simulink model "c00013M_harness"  (R2018a)
settings: Solver=FixedStepAuto  StartTime=0.0  StopTime=300  FixedStep=0.1  RelTol=1e-3
undefined symbols (not defined in the file): A1, hmax, PriorityTank, R1, R2, sigbuilder_block, TempThreshold
(part 8 of 93)

== system c00013M_harness/M022 ==
  note: VALUES
      | ---------------------------------
      | ControlType = 1 | 2 | 3
      | FillTank = 0 | 1
      | EmptyTank = 0 | 1
      | ManualReference between 0 and 1
      | Tempreature between 0 and 100
      | EmergencyButton = 0 | 1
      | LiquidLevel between 0 and 1 (hmax)
  note: Inputs For Tank2
  note: NAMES
      | --------------------------------------------
      | CT1 = ControlType Tank 1
      | F1 = Fill Tank 1
      | E1 = Empty Tank 1
      | MR1 = Manual Reference Tank1
      | T1 = Temperature Tank 1
      | EB1 = Emergency Button Tank 1
      | LL1 = Liquid Level 1
  note: Inputs For Tank3
  note: Inputs For Tank1
  CT1 : Inport
  T1 : Inport  Port=2
  EB1 : Inport  Port=3
  CT2 : Inport  Port=4
  F2 : Inport  Port=5
  E2 : Inport  Port=6
  MR2 : Inport  Port=7
  T2 : Inport  Port=8
  EB2 : Inport  Port=9
  CT3 : Inport  Port=10
  T3 : Inport  Port=11
  EB3 : Inport  Port=12
  Tank1 : Subsystem
  Tank2 : Subsystem
  Tank3 : Subsystem
  LL1 : Outport
  LL2 : Outport  Port=2
  LL3 : Outport  Port=3
  wires:
  EB1/1 -> Tank1/3(EB1)
  Tank2/1(LL2) -> LL2/1, Tank3/5(LL2), Tank1/4(LL2)
  Tank3/1(LL3) -> LL3/1, Tank2/8(LL3), Tank1/5(LL3)
  EB2/1 -> Tank2/6(EB2)
  CT2/1 -> Tank2/1(CT2)
  T1/1 -> Tank1/2(T1)
  Tank1/1(LL1) -> LL1/1, Tank3/4(LL1), Tank2/7(LL1)
  F2/1 -> Tank2/2(F2)
  E2/1 -> Tank2/3(E2)
  T2/1 -> Tank2/5(T2)
  CT3/1 -> Tank3/1(CT3)
  EB3/1 -> Tank3/3(EB3)
  T3/1 -> Tank3/2(T3)
  CT1/1 -> Tank1/1(CT1)
  MR2/1 -> Tank2/4(MR2)

== system c00013M_harness/M023 ==
  note: VALUES
      | ---------------------------------
      | ControlType = 1 | 2 | 3
      | FillTank = 0 | 1
      | EmptyTank = 0 | 1
      | ManualReference between 0 and 1
      | Tempreature between 0 and 100
      | EmergencyButton = 0 | 1
      | LiquidLevel between 0 and 1 (hmax)
  note: Inputs For Tank2
  note: NAMES
      | --------------------------------------------
      | CT1 = ControlType Tank 1
      | F1 = Fill Tank 1
      | E1 = Empty Tank 1
      | MR1 = Manual Reference Tank1
      | T1 = Temperature Tank 1
      | EB1 = Emergency Button Tank 1
      | LL1 = Liquid Level 1
  note: Inputs For Tank3
  note: Inputs For Tank1
  CT1 : Inport
  T1 : Inport  Port=2
  EB1 : Inport  Port=3
  CT2 : Inport  Port=4
  F2 : Inport  Port=5
  E2 : Inport  Port=6
  MR2 : Inport  Port=7
  T2 : Inport  Port=8
  EB2 : Inport  Port=9
  CT3 : Inport  Port=10
  T3 : Inport  Port=11
  EB3 : Inport  Port=12
  Tank1 : Subsystem
  Tank2 : Subsystem
  Tank3 : Subsystem
  LL1 : Outport
  LL2 : Outport  Port=2
  LL3 : Outport  Port=3
  wires:
  EB1/1 -> Tank1/3(EB1)
  Tank2/1(LL2) -> LL2/1, Tank3/5(LL2), Tank1/4(LL2)
  Tank3/1(LL3) -> LL3/1, Tank2/8(LL3), Tank1/5(LL3)
  EB2/1 -> Tank2/6(EB2)
  CT2/1 -> Tank2/1(CT2)
  T1/1 -> Tank1/2(T1)
  Tank1/1(LL1) -> LL1/1, Tank3/4(LL1), Tank2/7(LL1)
  F2/1 -> Tank2/2(F2)
  E2/1 -> Tank2/3(E2)
  T2/1 -> Tank2/5(T2)
  CT3/1 -> Tank3/1(CT3)
  EB3/1 -> Tank3/3(EB3)
  T3/1 -> Tank3/2(T3)
  CT1/1 -> Tank1/1(CT1)
  MR2/1 -> Tank2/4(MR2)

== system c00013M_harness/M024 ==
  note: VALUES
      | ---------------------------------
      | ControlType = 1 | 2 | 3
      | FillTank = 0 | 1
      | EmptyTank = 0 | 1
      | ManualReference between 0 and 1
      | Tempreature between 0 and 100
      | EmergencyButton = 0 | 1
      | LiquidLevel between 0 and 1 (hmax)
  note: Inputs For Tank2
  note: NAMES
      | --------------------------------------------
      | CT1 = ControlType Tank 1
      | F1 = Fill Tank 1
      | E1 = Empty Tank 1
      | MR1 = Manual Reference Tank1
      | T1 = Temperature Tank 1
      | EB1 = Emergency Button Tank 1
      | LL1 = Liquid Level 1
  note: Inputs For Tank3
  note: Inputs For Tank1
  CT1 : Inport
  T1 : Inport  Port=2
  EB1 : Inport  Port=3
  CT2 : Inport  Port=4
  F2 : Inport  Port=5
  E2 : Inport  Port=6
  MR2 : Inport  Port=7
  T2 : Inport  Port=8
  EB2 : Inport  Port=9
  CT3 : Inport  Port=10
  T3 : Inport  Port=11
  EB3 : Inport  Port=12
  Tank1 : Subsystem
  Tank2 : Subsystem
  Tank3 : Subsystem
  LL1 : Outport
  LL2 : Outport  Port=2
  LL3 : Outport  Port=3
  wires:
  EB1/1 -> Tank1/3(EB1)
  Tank2/1(LL2) -> LL2/1, Tank3/5(LL2), Tank1/4(LL2)
  Tank3/1(LL3) -> LL3/1, Tank2/8(LL3), Tank1/5(LL3)
  EB2/1 -> Tank2/6(EB2)
  CT2/1 -> Tank2/1(CT2)
  T1/1 -> Tank1/2(T1)
  Tank1/1(LL1) -> LL1/1, Tank3/4(LL1), Tank2/7(LL1)
  F2/1 -> Tank2/2(F2)
  E2/1 -> Tank2/3(E2)
  T2/1 -> Tank2/5(T2)
  CT3/1 -> Tank3/1(CT3)
  EB3/1 -> Tank3/3(EB3)
  T3/1 -> Tank3/2(T3)
  CT1/1 -> Tank1/1(CT1)
  MR2/1 -> Tank2/4(MR2)

== system c00013M_harness/M025 ==
  note: VALUES
      | ---------------------------------
      | ControlType = 1 | 2 | 3
      | FillTank = 0 | 1
      | EmptyTank = 0 | 1
      | ManualReference between 0 and 1
      | Tempreature between 0 and 100
      | EmergencyButton = 0 | 1
      | LiquidLevel between 0 and 1 (hmax)
  note: Inputs For Tank2
  note: NAMES
      | --------------------------------------------
      | CT1 = ControlType Tank 1
      | F1 = Fill Tank 1
      | E1 = Empty Tank 1
      | MR1 = Manual Reference Tank1
      | T1 = Temperature Tank 1
      | EB1 = Emergency Button Tank 1
      | LL1 = Liquid Level 1
  note: Inputs For Tank3
  note: Inputs For Tank1
  CT1 : Inport
  T1 : Inport  Port=2
  EB1 : Inport  Port=3
  CT2 : Inport  Port=4
  F2 : Inport  Port=5
  E2 : Inport  Port=6
  MR2 : Inport  Port=7
  T2 : Inport  Port=8
  EB2 : Inport  Port=9
  CT3 : Inport  Port=10
  T3 : Inport  Port=11
  EB3 : Inport  Port=12
  Tank1 : Subsystem
  Tank2 : Subsystem
  Tank3 : Subsystem
  LL1 : Outport
  LL2 : Outport  Port=2
  LL3 : Outport  Port=3
  wires:
  EB1/1 -> Tank1/3(EB1)
  Tank2/1(LL2) -> LL2/1, Tank3/5(LL2), Tank1/4(LL2)
  Tank3/1(LL3) -> LL3/1, Tank2/8(LL3), Tank1/5(LL3)
  EB2/1 -> Tank2/6(EB2)
  CT2/1 -> Tank2/1(CT2)
  T1/1 -> Tank1/2(T1)
  Tank1/1(LL1) -> LL1/1, Tank3/4(LL1), Tank2/7(LL1)
  F2/1 -> Tank2/2(F2)
  E2/1 -> Tank2/3(E2)
  T2/1 -> Tank2/5(T2)
  CT3/1 -> Tank3/1(CT3)
  EB3/1 -> Tank3/3(EB3)
  T3/1 -> Tank3/2(T3)
  CT1/1 -> Tank1/1(CT1)
  MR2/1 -> Tank2/4(MR2)

== system c00013M_harness/M026 ==
  note: VALUES
      | ---------------------------------
      | ControlType = 1 | 2 | 3
      | FillTank = 0 | 1
      | EmptyTank = 0 | 1
      | ManualReference between 0 and 1
      | Tempreature between 0 and 100
      | EmergencyButton = 0 | 1
      | LiquidLevel between 0 and 1 (hmax)
  note: Inputs For Tank2
  note: NAMES
      | --------------------------------------------
      | CT1 = ControlType Tank 1
      | F1 = Fill Tank 1
      | E1 = Empty Tank 1
      | MR1 = Manual Reference Tank1
      | T1 = Temperature Tank 1
      | EB1 = Emergency Button Tank 1
      | LL1 = Liquid Level 1
  note: Inputs For Tank3
  note: Inputs For Tank1
  CT1 : Inport
  T1 : Inport  Port=2
  EB1 : Inport  Port=3
  CT2 : Inport  Port=4
  F2 : Inport  Port=5
  E2 : Inport  Port=6
  MR2 : Inport  Port=7
  T2 : Inport  Port=8
  EB2 : Inport  Port=9
  CT3 : Inport  Port=10
  T3 : Inport  Port=11
  EB3 : Inport  Port=12
  Tank1 : Subsystem
  Tank2 : Subsystem
  Tank3 : Subsystem
  LL1 : Outport
  LL2 : Outport  Port=2
  LL3 : Outport  Port=3
  wires:
  EB1/1 -> Tank1/3(EB1)
  Tank2/1(LL2) -> LL2/1, Tank3/5(LL2), Tank1/4(LL2)
  Tank3/1(LL3) -> LL3/1, Tank2/8(LL3), Tank1/5(LL3)
  EB2/1 -> Tank2/6(EB2)
  CT2/1 -> Tank2/1(CT2)
  T1/1 -> Tank1/2(T1)
  Tank1/1(LL1) -> LL1/1, Tank3/4(LL1), Tank2/7(LL1)
  F2/1 -> Tank2/2(F2)
  E2/1 -> Tank2/3(E2)
  T2/1 -> Tank2/5(T2)
  CT3/1 -> Tank3/1(CT3)
  EB3/1 -> Tank3/3(EB3)
  T3/1 -> Tank3/2(T3)
  CT1/1 -> Tank1/1(CT1)
  MR2/1 -> Tank2/4(MR2)

== system c00013M_harness/M027 ==
  note: VALUES
      | ---------------------------------
      | ControlType = 1 | 2 | 3
      | FillTank = 0 | 1
      | EmptyTank = 0 | 1
      | ManualReference between 0 and 1
      | Tempreature between 0 and 100
      | EmergencyButton = 0 | 1
      | LiquidLevel between 0 and 1 (hmax)
  note: Inputs For Tank2
  note: NAMES
      | --------------------------------------------
      | CT1 = ControlType Tank 1
      | F1 = Fill Tank 1
      | E1 = Empty Tank 1
      | MR1 = Manual Reference Tank1
      | T1 = Temperature Tank 1
      | EB1 = Emergency Button Tank 1
      | LL1 = Liquid Level 1
  note: Inputs For Tank3
  note: Inputs For Tank1
  CT1 : Inport
  T1 : Inport  Port=2
  EB1 : Inport  Port=3
  CT2 : Inport  Port=4
  F2 : Inport  Port=5
  E2 : Inport  Port=6
  MR2 : Inport  Port=7
  T2 : Inport  Port=8
  EB2 : Inport  Port=9
  CT3 : Inport  Port=10
  T3 : Inport  Port=11
  EB3 : Inport  Port=12
  Tank1 : Subsystem
  Tank2 : Subsystem
  Tank3 : Subsystem
  LL1 : Outport
  LL2 : Outport  Port=2
  LL3 : Outport  Port=3
  wires:
  EB1/1 -> Tank1/3(EB1)
  Tank2/1(LL2) -> LL2/1, Tank3/5(LL2), Tank1/4(LL2)
  Tank3/1(LL3) -> LL3/1, Tank2/8(LL3), Tank1/5(LL3)
  EB2/1 -> Tank2/6(EB2)
  CT2/1 -> Tank2/1(CT2)
  T1/1 -> Tank1/2(T1)
  Tank1/1(LL1) -> LL1/1, Tank3/4(LL1), Tank2/7(LL1)
  F2/1 -> Tank2/2(F2)
  E2/1 -> Tank2/3(E2)
  T2/1 -> Tank2/5(T2)
  CT3/1 -> Tank3/1(CT3)
  EB3/1 -> Tank3/3(EB3)
  T3/1 -> Tank3/2(T3)
  CT1/1 -> Tank1/1(CT1)
  MR2/1 -> Tank2/4(MR2)

== system c00013M_harness/M028 ==
  note: VALUES
      | ---------------------------------
      | ControlType = 1 | 2 | 3
      | FillTank = 0 | 1
      | EmptyTank = 0 | 1
      | ManualReference between 0 and 1
      | Tempreature between 0 and 100
      | EmergencyButton = 0 | 1
      | LiquidLevel between 0 and 1 (hmax)
  note: Inputs For Tank2
  note: NAMES
      | --------------------------------------------
      | CT1 = ControlType Tank 1
      | F1 = Fill Tank 1
      | E1 = Empty Tank 1
      | MR1 = Manual Reference Tank1
      | T1 = Temperature Tank 1
      | EB1 = Emergency Button Tank 1
      | LL1 = Liquid Level 1
  note: Inputs For Tank3
  note: Inputs For Tank1
  CT1 : Inport
  T1 : Inport  Port=2
  EB1 : Inport  Port=3
  CT2 : Inport  Port=4
  F2 : Inport  Port=5
  E2 : Inport  Port=6
  MR2 : Inport  Port=7
  T2 : Inport  Port=8
  EB2 : Inport  Port=9
  CT3 : Inport  Port=10
  T3 : Inport  Port=11
  EB3 : Inport  Port=12
  Tank1 : Subsystem
  Tank2 : Subsystem
  Tank3 : Subsystem
  LL1 : Outport
  LL2 : Outport  Port=2
  LL3 : Outport  Port=3
  wires:
  EB1/1 -> Tank1/3(EB1)
  Tank2/1(LL2) -> LL2/1, Tank3/5(LL2), Tank1/4(LL2)
  Tank3/1(LL3) -> LL3/1, Tank2/8(LL3), Tank1/5(LL3)
  EB2/1 -> Tank2/6(EB2)
  CT2/1 -> Tank2/1(CT2)
  T1/1 -> Tank1/2(T1)
  Tank1/1(LL1) -> LL1/1, Tank3/4(LL1), Tank2/7(LL1)
  F2/1 -> Tank2/2(F2)
  E2/1 -> Tank2/3(E2)
  T2/1 -> Tank2/5(T2)
  CT3/1 -> Tank3/1(CT3)
  EB3/1 -> Tank3/3(EB3)
  T3/1 -> Tank3/2(T3)
  CT1/1 -> Tank1/1(CT1)
  MR2/1 -> Tank2/4(MR2)

== system c00013M_harness/M029 ==
  note: VALUES
      | ---------------------------------
      | ControlType = 1 | 2 | 3
      | FillTank = 0 | 1
      | EmptyTank = 0 | 1
      | ManualReference between 0 and 1
      | Tempreature between 0 and 100
      | EmergencyButton = 0 | 1
      | LiquidLevel between 0 and 1 (hmax)
  note: Inputs For Tank2
  note: NAMES
      | --------------------------------------------
      | CT1 = ControlType Tank 1
      | F1 = Fill Tank 1
      | E1 = Empty Tank 1
      | MR1 = Manual Reference Tank1
      | T1 = Temperature Tank 1
      | EB1 = Emergency Button Tank 1
      | LL1 = Liquid Level 1
  note: Inputs For Tank3
  note: Inputs For Tank1
  CT1 : Inport
  T1 : Inport  Port=2
  EB1 : Inport  Port=3
  CT2 : Inport  Port=4
  F2 : Inport  Port=5
  E2 : Inport  Port=6
  MR2 : Inport  Port=7
  T2 : Inport  Port=8
  EB2 : Inport  Port=9
  CT3 : Inport  Port=10
  T3 : Inport  Port=11
  EB3 : Inport  Port=12
  Tank1 : Subsystem
  Tank2 : Subsystem
  Tank3 : Subsystem
  LL1 : Outport
  LL2 : Outport  Port=2
  LL3 : Outport  Port=3
  wires:
  EB1/1 -> Tank1/3(EB1)
  Tank2/1(LL2) -> LL2/1, Tank3/5(LL2), Tank1/4(LL2)
  Tank3/1(LL3) -> LL3/1, Tank2/8(LL3), Tank1/5(LL3)
  EB2/1 -> Tank2/6(EB2)
  CT2/1 -> Tank2/1(CT2)
  T1/1 -> Tank1/2(T1)
  Tank1/1(LL1) -> LL1/1, Tank3/4(LL1), Tank2/7(LL1)
  F2/1 -> Tank2/2(F2)
  E2/1 -> Tank2/3(E2)
  T2/1 -> Tank2/5(T2)
  CT3/1 -> Tank3/1(CT3)
  EB3/1 -> Tank3/3(EB3)
  T3/1 -> Tank3/2(T3)
  CT1/1 -> Tank1/1(CT1)
  MR2/1 -> Tank2/4(MR2)

== system c00013M_harness/M030 ==
  note: VALUES
      | ---------------------------------
      | ControlType = 1 | 2 | 3
      | FillTank = 0 | 1
      | EmptyTank = 0 | 1
      | ManualReference between 0 and 1
      | Tempreature between 0 and 100
      | EmergencyButton = 0 | 1
      | LiquidLevel between 0 and 1 (hmax)
  note: Inputs For Tank2
  note: NAMES
      | --------------------------------------------
      | CT1 = ControlType Tank 1
      | F1 = Fill Tank 1
      | E1 = Empty Tank 1
      | MR1 = Manual Reference Tank1
      | T1 = Temperature Tank 1
      | EB1 = Emergency Button Tank 1
      | LL1 = Liquid Level 1
  note: Inputs For Tank3
  note: Inputs For Tank1
  CT1 : Inport
  T1 : Inport  Port=2
  EB1 : Inport  Port=3
  CT2 : Inport  Port=4
  F2 : Inport  Port=5
  E2 : Inport  Port=6
  MR2 : Inport  Port=7
  T2 : Inport  Port=8
  EB2 : Inport  Port=9
  CT3 : Inport  Port=10
  T3 : Inport  Port=11
  EB3 : Inport  Port=12
  Tank1 : Subsystem
  Tank2 : Subsystem
  Tank3 : Subsystem
  LL1 : Outport
  LL2 : Outport  Port=2
  LL3 : Outport  Port=3
  wires:
  EB1/1 -> Tank1/3(EB1)
  Tank2/1(LL2) -> LL2/1, Tank3/5(LL2), Tank1/4(LL2)
  Tank3/1(LL3) -> LL3/1, Tank2/8(LL3), Tank1/5(LL3)
  EB2/1 -> Tank2/6(EB2)
  CT2/1 -> Tank2/1(CT2)
  T1/1 -> Tank1/2(T1)
  Tank1/1(LL1) -> LL1/1, Tank3/4(LL1), Tank2/7(LL1)
  F2/1 -> Tank2/2(F2)
  E2/1 -> Tank2/3(E2)
  T2/1 -> Tank2/5(T2)
  CT3/1 -> Tank3/1(CT3)
  EB3/1 -> Tank3/3(EB3)
  T3/1 -> Tank3/2(T3)
  CT1/1 -> Tank1/1(CT1)
  MR2/1 -> Tank2/4(MR2)

== system c00013M_harness/M031 ==
  note: VALUES
      | ---------------------------------
      | ControlType = 1 | 2 | 3
      | FillTank = 0 | 1
      | EmptyTank = 0 | 1
      | ManualReference between 0 and 1
      | Tempreature between 0 and 100
      | EmergencyButton = 0 | 1
      | LiquidLevel between 0 and 1 (hmax)
  note: Inputs For Tank2
  note: NAMES
      | --------------------------------------------
      | CT1 = ControlType Tank 1
      | F1 = Fill Tank 1
      | E1 = Empty Tank 1
      | MR1 = Manual Reference Tank1
      | T1 = Temperature Tank 1
      | EB1 = Emergency Button Tank 1
      | LL1 = Liquid Level 1
  note: Inputs For Tank3
  note: Inputs For Tank1
  CT1 : Inport
  T1 : Inport  Port=2
  EB1 : Inport  Port=3
  CT2 : Inport  Port=4
  F2 : Inport  Port=5
  E2 : Inport  Port=6
  MR2 : Inport  Port=7
  T2 : Inport  Port=8
  EB2 : Inport  Port=9
  CT3 : Inport  Port=10
  T3 : Inport  Port=11
  EB3 : Inport  Port=12
  Tank1 : Subsystem
  Tank2 : Subsystem
  Tank3 : Subsystem
  LL1 : Outport
  LL2 : Outport  Port=2
  LL3 : Outport  Port=3
  wires:
  EB1/1 -> Tank1/3(EB1)
  Tank2/1(LL2) -> LL2/1, Tank3/5(LL2), Tank1/4(LL2)
  Tank3/1(LL3) -> LL3/1, Tank2/8(LL3), Tank1/5(LL3)
  EB2/1 -> Tank2/6(EB2)
  CT2/1 -> Tank2/1(CT2)
  T1/1 -> Tank1/2(T1)
  Tank1/1(LL1) -> LL1/1, Tank3/4(LL1), Tank2/7(LL1)
  F2/1 -> Tank2/2(F2)
  E2/1 -> Tank2/3(E2)
  T2/1 -> Tank2/5(T2)
  CT3/1 -> Tank3/1(CT3)
  EB3/1 -> Tank3/3(EB3)
  T3/1 -> Tank3/2(T3)
  CT1/1 -> Tank1/1(CT1)
  MR2/1 -> Tank2/4(MR2)

== system c00013M_harness/M032 ==
  note: VALUES
      | ---------------------------------
      | ControlType = 1 | 2 | 3
      | FillTank = 0 | 1
      | EmptyTank = 0 | 1
      | ManualReference between 0 and 1
      | Tempreature between 0 and 100
      | EmergencyButton = 0 | 1
      | LiquidLevel between 0 and 1 (hmax)
  note: Inputs For Tank2
  note: NAMES
      | --------------------------------------------
      | CT1 = ControlType Tank 1
      | F1 = Fill Tank 1
      | E1 = Empty Tank 1
      | MR1 = Manual Reference Tank1
      | T1 = Temperature Tank 1
      | EB1 = Emergency Button Tank 1
      | LL1 = Liquid Level 1
  note: Inputs For Tank3
  note: Inputs For Tank1
  CT1 : Inport
  T1 : Inport  Port=2
  EB1 : Inport  Port=3
  CT2 : Inport  Port=4
  F2 : Inport  Port=5
  E2 : Inport  Port=6
  MR2 : Inport  Port=7
  T2 : Inport  Port=8
  EB2 : Inport  Port=9
  CT3 : Inport  Port=10
  T3 : Inport  Port=11
  EB3 : Inport  Port=12
  Tank1 : Subsystem
  Tank2 : Subsystem
  Tank3 : Subsystem
  LL1 : Outport
  LL2 : Outport  Port=2
  LL3 : Outport  Port=3
  wires:
  EB1/1 -> Tank1/3(EB1)
  Tank2/1(LL2) -> LL2/1, Tank3/5(LL2), Tank1/4(LL2)
  Tank3/1(LL3) -> LL3/1, Tank2/8(LL3), Tank1/5(LL3)
  EB2/1 -> Tank2/6(EB2)
  CT2/1 -> Tank2/1(CT2)
  T1/1 -> Tank1/2(T1)
  Tank1/1(LL1) -> LL1/1, Tank3/4(LL1), Tank2/7(LL1)
  F2/1 -> Tank2/2(F2)
  E2/1 -> Tank2/3(E2)
  T2/1 -> Tank2/5(T2)
  CT3/1 -> Tank3/1(CT3)
  EB3/1 -> Tank3/3(EB3)
  T3/1 -> Tank3/2(T3)
  CT1/1 -> Tank1/1(CT1)
  MR2/1 -> Tank2/4(MR2)

== system c00013M_harness/M033 ==
  note: VALUES
      | ---------------------------------
      | ControlType = 1 | 2 | 3
      | FillTank = 0 | 1
      | EmptyTank = 0 | 1
      | ManualReference between 0 and 1
      | Tempreature between 0 and 100
      | EmergencyButton = 0 | 1
      | LiquidLevel between 0 and 1 (hmax)
  note: Inputs For Tank2
  note: NAMES
      | --------------------------------------------
      | CT1 = ControlType Tank 1
      | F1 = Fill Tank 1
      | E1 = Empty Tank 1
      | MR1 = Manual Reference Tank1
      | T1 = Temperature Tank 1
      | EB1 = Emergency Button Tank 1
      | LL1 = Liquid Level 1
  note: Inputs For Tank3
  note: Inputs For Tank1
  CT1 : Inport
  T1 : Inport  Port=2
  EB1 : Inport  Port=3
  CT2 : Inport  Port=4
  F2 : Inport  Port=5
  E2 : Inport  Port=6
  MR2 : Inport  Port=7
  T2 : Inport  Port=8
  EB2 : Inport  Port=9
  CT3 : Inport  Port=10
  T3 : Inport  Port=11
  EB3 : Inport  Port=12
  Tank1 : Subsystem
  Tank2 : Subsystem
  Tank3 : Subsystem
  LL1 : Outport
  LL2 : Outport  Port=2
  LL3 : Outport  Port=3
  wires:
  EB1/1 -> Tank1/3(EB1)
  Tank2/1(LL2) -> LL2/1, Tank3/5(LL2), Tank1/4(LL2)
  Tank3/1(LL3) -> LL3/1, Tank2/8(LL3), Tank1/5(LL3)
  EB2/1 -> Tank2/6(EB2)
  CT2/1 -> Tank2/1(CT2)
  T1/1 -> Tank1/2(T1)
  Tank1/1(LL1) -> LL1/1, Tank3/4(LL1), Tank2/7(LL1)
  F2/1 -> Tank2/2(F2)
  E2/1 -> Tank2/3(E2)
  T2/1 -> Tank2/5(T2)
  CT3/1 -> Tank3/1(CT3)
  EB3/1 -> Tank3/3(EB3)
  T3/1 -> Tank3/2(T3)
  CT1/1 -> Tank1/1(CT1)
  MR2/1 -> Tank2/4(MR2)

== system c00013M_harness/M034 ==
  note: VALUES
      | ---------------------------------
      | ControlType = 1 | 2 | 3
      | FillTank = 0 | 1
      | EmptyTank = 0 | 1
      | ManualReference between 0 and 1
      | Tempreature between 0 and 100
      | EmergencyButton = 0 | 1
      | LiquidLevel between 0 and 1 (hmax)
  note: Inputs For Tank2
  note: NAMES
      | --------------------------------------------
      | CT1 = ControlType Tank 1
      | F1 = Fill Tank 1
      | E1 = Empty Tank 1
      | MR1 = Manual Reference Tank1
      | T1 = Temperature Tank 1
      | EB1 = Emergency Button Tank 1
      | LL1 = Liquid Level 1
  note: Inputs For Tank3
  note: Inputs For Tank1
  CT1 : Inport
  T1 : Inport  Port=2
  EB1 : Inport  Port=3
  CT2 : Inport  Port=4
  F2 : Inport  Port=5
  E2 : Inport  Port=6
  MR2 : Inport  Port=7
  T2 : Inport  Port=8
  EB2 : Inport  Port=9
  CT3 : Inport  Port=10
  T3 : Inport  Port=11
  EB3 : Inport  Port=12
  Tank1 : Subsystem
  Tank2 : Subsystem
  Tank3 : Subsystem
  LL1 : Outport
  LL2 : Outport  Port=2
  LL3 : Outport  Port=3
  wires:
  EB1/1 -> Tank1/3(EB1)
  Tank2/1(LL2) -> LL2/1, Tank3/5(LL2), Tank1/4(LL2)
  Tank3/1(LL3) -> LL3/1, Tank2/8(LL3), Tank1/5(LL3)
  EB2/1 -> Tank2/6(EB2)
  CT2/1 -> Tank2/1(CT2)
  T1/1 -> Tank1/2(T1)
  Tank1/1(LL1) -> LL1/1, Tank3/4(LL1), Tank2/7(LL1)
  F2/1 -> Tank2/2(F2)
  E2/1 -> Tank2/3(E2)
  T2/1 -> Tank2/5(T2)
  CT3/1 -> Tank3/1(CT3)
  EB3/1 -> Tank3/3(EB3)
  T3/1 -> Tank3/2(T3)
  CT1/1 -> Tank1/1(CT1)
  MR2/1 -> Tank2/4(MR2)

== system c00013M_harness/M035 ==
  note: VALUES
      | ---------------------------------
      | ControlType = 1 | 2 | 3
      | FillTank = 0 | 1
      | EmptyTank = 0 | 1
      | ManualReference between 0 and 1
      | Tempreature between 0 and 100
      | EmergencyButton = 0 | 1
      | LiquidLevel between 0 and 1 (hmax)
  note: Inputs For Tank2
  note: NAMES
      | --------------------------------------------
      | CT1 = ControlType Tank 1
      | F1 = Fill Tank 1
      | E1 = Empty Tank 1
      | MR1 = Manual Reference Tank1
      | T1 = Temperature Tank 1
      | EB1 = Emergency Button Tank 1
      | LL1 = Liquid Level 1
  note: Inputs For Tank3
  note: Inputs For Tank1
  CT1 : Inport
  T1 : Inport  Port=2
  EB1 : Inport  Port=3
  CT2 : Inport  Port=4
  F2 : Inport  Port=5
  E2 : Inport  Port=6
  MR2 : Inport  Port=7
  T2 : Inport  Port=8
  EB2 : Inport  Port=9
  CT3 : Inport  Port=10
  T3 : Inport  Port=11
  EB3 : Inport  Port=12
  Tank1 : Subsystem
  Tank2 : Subsystem
  Tank3 : Subsystem
  LL1 : Outport
  LL2 : Outport  Port=2
  LL3 : Outport  Port=3
  wires:
  EB1/1 -> Tank1/3(EB1)
  Tank2/1(LL2) -> LL2/1, Tank3/5(LL2), Tank1/4(LL2)
  Tank3/1(LL3) -> LL3/1, Tank2/8(LL3), Tank1/5(LL3)
  EB2/1 -> Tank2/6(EB2)
  CT2/1 -> Tank2/1(CT2)
  T1/1 -> Tank1/2(T1)
  Tank1/1(LL1) -> LL1/1, Tank3/4(LL1), Tank2/7(LL1)
  F2/1 -> Tank2/2(F2)
  E2/1 -> Tank2/3(E2)
  T2/1 -> Tank2/5(T2)
  CT3/1 -> Tank3/1(CT3)
  EB3/1 -> Tank3/3(EB3)
  T3/1 -> Tank3/2(T3)
  CT1/1 -> Tank1/1(CT1)
  MR2/1 -> Tank2/4(MR2)

== system c00013M_harness/M057 ==
  note: VALUES
      | ---------------------------------
      | ControlType = 1 | 2 | 3
      | FillTank = 0 | 1
      | EmptyTank = 0 | 1
      | ManualReference between 0 and 1
      | Tempreature between 0 and 100
      | EmergencyButton = 0 | 1
      | LiquidLevel between 0 and 1 (hmax)
  note: Inputs For Tank2
  note: NAMES
      | --------------------------------------------
      | CT1 = ControlType Tank 1
      | F1 = Fill Tank 1
      | E1 = Empty Tank 1
      | MR1 = Manual Reference Tank1
      | T1 = Temperature Tank 1
      | EB1 = Emergency Button Tank 1
      | LL1 = Liquid Level 1
  note: Inputs For Tank3
  note: Inputs For Tank1
  CT1 : Inport
  T1 : Inport  Port=2
  EB1 : Inport  Port=3
  CT2 : Inport  Port=4
  F2 : Inport  Port=5
  E2 : Inport  Port=6
  MR2 : Inport  Port=7
  T2 : Inport  Port=8
  EB2 : Inport  Port=9
  CT3 : Inport  Port=10
  T3 : Inport  Port=11
  EB3 : Inport  Port=12
  Tank1 : Subsystem
  Tank2 : Subsystem
  Tank3 : Subsystem
  LL1 : Outport
  LL2 : Outport  Port=2
  LL3 : Outport  Port=3
  wires:
  EB1/1 -> Tank1/3(EB1)
  Tank2/1(LL2) -> LL2/1, Tank3/5(LL2), Tank1/4(LL2)
  Tank3/1(LL3) -> LL3/1, Tank2/8(LL3), Tank1/5(LL3)
  EB2/1 -> Tank2/6(EB2)
  CT2/1 -> Tank2/1(CT2)
  T1/1 -> Tank1/2(T1)
  Tank1/1(LL1) -> LL1/1, Tank3/4(LL1), Tank2/7(LL1)
  F2/1 -> Tank2/2(F2)
  E2/1 -> Tank2/3(E2)
  T2/1 -> Tank2/5(T2)
  CT3/1 -> Tank3/1(CT3)
  EB3/1 -> Tank3/3(EB3)
  T3/1 -> Tank3/2(T3)
  CT1/1 -> Tank1/1(CT1)
  MR2/1 -> Tank2/4(MR2)

== system c00013M_harness/M058 ==
  note: VALUES
      | ---------------------------------
      | ControlType = 1 | 2 | 3
      | FillTank = 0 | 1
      | EmptyTank = 0 | 1
      | ManualReference between 0 and 1
      | Tempreature between 0 and 100
      | EmergencyButton = 0 | 1
      | LiquidLevel between 0 and 1 (hmax)
  note: Inputs For Tank2
  note: NAMES
      | --------------------------------------------
      | CT1 = ControlType Tank 1
      | F1 = Fill Tank 1
      | E1 = Empty Tank 1
      | MR1 = Manual Reference Tank1
      | T1 = Temperature Tank 1
      | EB1 = Emergency Button Tank 1
      | LL1 = Liquid Level 1
  note: Inputs For Tank3
  note: Inputs For Tank1
  CT1 : Inport
  T1 : Inport  Port=2
  EB1 : Inport  Port=3
  CT2 : Inport  Port=4
  F2 : Inport  Port=5
  E2 : Inport  Port=6
  MR2 : Inport  Port=7
  T2 : Inport  Port=8
  EB2 : Inport  Port=9
  CT3 : Inport  Port=10
  T3 : Inport  Port=11
  EB3 : Inport  Port=12
  Tank1 : Subsystem
  Tank2 : Subsystem
  Tank3 : Subsystem
  LL1 : Outport
  LL2 : Outport  Port=2
  LL3 : Outport  Port=3
  wires:
  EB1/1 -> Tank1/3(EB1)
  Tank2/1(LL2) -> LL2/1, Tank3/5(LL2), Tank1/4(LL2)
  Tank3/1(LL3) -> LL3/1, Tank2/8(LL3), Tank1/5(LL3)
  EB2/1 -> Tank2/6(EB2)
  CT2/1 -> Tank2/1(CT2)
  T1/1 -> Tank1/2(T1)
  Tank1/1(LL1) -> LL1/1, Tank3/4(LL1), Tank2/7(LL1)
  F2/1 -> Tank2/2(F2)
  E2/1 -> Tank2/3(E2)
  T2/1 -> Tank2/5(T2)
  CT3/1 -> Tank3/1(CT3)
  EB3/1 -> Tank3/3(EB3)
  T3/1 -> Tank3/2(T3)
  CT1/1 -> Tank1/1(CT1)
  MR2/1 -> Tank2/4(MR2)

== system c00013M_harness/M059 ==
  note: VALUES
      | ---------------------------------
      | ControlType = 1 | 2 | 3
      | FillTank = 0 | 1
      | EmptyTank = 0 | 1
      | ManualReference between 0 and 1
      | Tempreature between 0 and 100
      | EmergencyButton = 0 | 1
      | LiquidLevel between 0 and 1 (hmax)
  note: Inputs For Tank2
  note: NAMES
      | --------------------------------------------
      | CT1 = ControlType Tank 1
      | F1 = Fill Tank 1
      | E1 = Empty Tank 1
      | MR1 = Manual Reference Tank1
      | T1 = Temperature Tank 1
      | EB1 = Emergency Button Tank 1
      | LL1 = Liquid Level 1
  note: Inputs For Tank3
  note: Inputs For Tank1
  CT1 : Inport
  T1 : Inport  Port=2
  EB1 : Inport  Port=3
  CT2 : Inport  Port=4
  F2 : Inport  Port=5
  E2 : Inport  Port=6
  MR2 : Inport  Port=7
  T2 : Inport  Port=8
  EB2 : Inport  Port=9
  CT3 : Inport  Port=10
  T3 : Inport  Port=11
  EB3 : Inport  Port=12
  Tank1 : Subsystem
  Tank2 : Subsystem
  Tank3 : Subsystem
  LL1 : Outport
  LL2 : Outport  Port=2
  LL3 : Outport  Port=3
  wires:
  EB1/1 -> Tank1/3(EB1)
  Tank2/1(LL2) -> LL2/1, Tank3/5(LL2), Tank1/4(LL2)
  Tank3/1(LL3) -> LL3/1, Tank2/8(LL3), Tank1/5(LL3)
  EB2/1 -> Tank2/6(EB2)
  CT2/1 -> Tank2/1(CT2)
  T1/1 -> Tank1/2(T1)
  Tank1/1(LL1) -> LL1/1, Tank3/4(LL1), Tank2/7(LL1)
  F2/1 -> Tank2/2(F2)
  E2/1 -> Tank2/3(E2)
  T2/1 -> Tank2/5(T2)
  CT3/1 -> Tank3/1(CT3)
  EB3/1 -> Tank3/3(EB3)
  T3/1 -> Tank3/2(T3)
  CT1/1 -> Tank1/1(CT1)
  MR2/1 -> Tank2/4(MR2)

== system c00013M_harness/M060 ==
  note: VALUES
      | ---------------------------------
      | ControlType = 1 | 2 | 3
      | FillTank = 0 | 1
      | EmptyTank = 0 | 1
      | ManualReference between 0 and 1
      | Tempreature between 0 and 100
      | EmergencyButton = 0 | 1
      | LiquidLevel between 0 and 1 (hmax)
  note: Inputs For Tank2
  note: NAMES
      | --------------------------------------------
      | CT1 = ControlType Tank 1
      | F1 = Fill Tank 1
      | E1 = Empty Tank 1
      | MR1 = Manual Reference Tank1
      | T1 = Temperature Tank 1
      | EB1 = Emergency Button Tank 1
      | LL1 = Liquid Level 1
  note: Inputs For Tank3
  note: Inputs For Tank1
  CT1 : Inport
  T1 : Inport  Port=2
  EB1 : Inport  Port=3
  CT2 : Inport  Port=4
  F2 : Inport  Port=5
  E2 : Inport  Port=6
  MR2 : Inport  Port=7
  T2 : Inport  Port=8
  EB2 : Inport  Port=9
  CT3 : Inport  Port=10
  T3 : Inport  Port=11
  EB3 : Inport  Port=12
  Tank1 : Subsystem
  Tank2 : Subsystem
  Tank3 : Subsystem
  LL1 : Outport
  LL2 : Outport  Port=2
  LL3 : Outport  Port=3
  wires:
  EB1/1 -> Tank1/3(EB1)
  Tank2/1(LL2) -> LL2/1, Tank3/5(LL2), Tank1/4(LL2)
  Tank3/1(LL3) -> LL3/1, Tank2/8(LL3), Tank1/5(LL3)
  EB2/1 -> Tank2/6(EB2)
  CT2/1 -> Tank2/1(CT2)
  T1/1 -> Tank1/2(T1)
  Tank1/1(LL1) -> LL1/1, Tank3/4(LL1), Tank2/7(LL1)
  F2/1 -> Tank2/2(F2)
  E2/1 -> Tank2/3(E2)
  T2/1 -> Tank2/5(T2)
  CT3/1 -> Tank3/1(CT3)
  EB3/1 -> Tank3/3(EB3)
  T3/1 -> Tank3/2(T3)
  CT1/1 -> Tank1/1(CT1)
  MR2/1 -> Tank2/4(MR2)

== system c00013M_harness/M061 ==
  note: VALUES
      | ---------------------------------
      | ControlType = 1 | 2 | 3
      | FillTank = 0 | 1
      | EmptyTank = 0 | 1
      | ManualReference between 0 and 1
      | Tempreature between 0 and 100
      | EmergencyButton = 0 | 1
      | LiquidLevel between 0 and 1 (hmax)
  note: Inputs For Tank2
  note: NAMES
      | --------------------------------------------
      | CT1 = ControlType Tank 1
      | F1 = Fill Tank 1
      | E1 = Empty Tank 1
      | MR1 = Manual Reference Tank1
      | T1 = Temperature Tank 1
      | EB1 = Emergency Button Tank 1
      | LL1 = Liquid Level 1
  note: Inputs For Tank3
  note: Inputs For Tank1
  CT1 : Inport
  T1 : Inport  Port=2
  EB1 : Inport  Port=3
  CT2 : Inport  Port=4
  F2 : Inport  Port=5
  E2 : Inport  Port=6
  MR2 : Inport  Port=7
  T2 : Inport  Port=8
  EB2 : Inport  Port=9
  CT3 : Inport  Port=10
  T3 : Inport  Port=11
  EB3 : Inport  Port=12
  Tank1 : Subsystem
  Tank2 : Subsystem
  Tank3 : Subsystem
  LL1 : Outport
  LL2 : Outport  Port=2
  LL3 : Outport  Port=3
  wires:
  EB1/1 -> Tank1/3(EB1)
  Tank2/1(LL2) -> LL2/1, Tank3/5(LL2), Tank1/4(LL2)
  Tank3/1(LL3) -> LL3/1, Tank2/8(LL3), Tank1/5(LL3)
  EB2/1 -> Tank2/6(EB2)
  CT2/1 -> Tank2/1(CT2)
  T1/1 -> Tank1/2(T1)
  Tank1/1(LL1) -> LL1/1, Tank3/4(LL1), Tank2/7(LL1)
  F2/1 -> Tank2/2(F2)
  E2/1 -> Tank2/3(E2)
  T2/1 -> Tank2/5(T2)
  CT3/1 -> Tank3/1(CT3)
  EB3/1 -> Tank3/3(EB3)
  T3/1 -> Tank3/2(T3)
  CT1/1 -> Tank1/1(CT1)
  MR2/1 -> Tank2/4(MR2)

== system c00013M_harness/M062 ==
  note: VALUES
      | ---------------------------------
      | ControlType = 1 | 2 | 3
      | FillTank = 0 | 1
      | EmptyTank = 0 | 1
      | ManualReference between 0 and 1
      | Tempreature between 0 and 100
      | EmergencyButton = 0 | 1
      | LiquidLevel between 0 and 1 (hmax)
  note: Inputs For Tank2
  note: NAMES
      | --------------------------------------------
      | CT1 = ControlType Tank 1
      | F1 = Fill Tank 1
      | E1 = Empty Tank 1
      | MR1 = Manual Reference Tank1
      | T1 = Temperature Tank 1
      | EB1 = Emergency Button Tank 1
      | LL1 = Liquid Level 1
  note: Inputs For Tank3
  note: Inputs For Tank1
  CT1 : Inport
  T1 : Inport  Port=2
  EB1 : Inport  Port=3
  CT2 : Inport  Port=4
  F2 : Inport  Port=5
  E2 : Inport  Port=6
  MR2 : Inport  Port=7
  T2 : Inport  Port=8
  EB2 : Inport  Port=9
  CT3 : Inport  Port=10
  T3 : Inport  Port=11
  EB3 : Inport  Port=12
  Tank1 : Subsystem
  Tank2 : Subsystem
  Tank3 : Subsystem
  LL1 : Outport
  LL2 : Outport  Port=2
  LL3 : Outport  Port=3
  wires:
  EB1/1 -> Tank1/3(EB1)
  Tank2/1(LL2) -> LL2/1, Tank3/5(LL2), Tank1/4(LL2)
  Tank3/1(LL3) -> LL3/1, Tank2/8(LL3), Tank1/5(LL3)
  EB2/1 -> Tank2/6(EB2)
  CT2/1 -> Tank2/1(CT2)
  T1/1 -> Tank1/2(T1)
  Tank1/1(LL1) -> LL1/1, Tank3/4(LL1), Tank2/7(LL1)
  F2/1 -> Tank2/2(F2)
  E2/1 -> Tank2/3(E2)
  T2/1 -> Tank2/5(T2)
  CT3/1 -> Tank3/1(CT3)
  EB3/1 -> Tank3/3(EB3)
  T3/1 -> Tank3/2(T3)
  CT1/1 -> Tank1/1(CT1)
  MR2/1 -> Tank2/4(MR2)

== system c00013M_harness/M063 ==
  note: VALUES
      | ---------------------------------
      | ControlType = 1 | 2 | 3
      | FillTank = 0 | 1
      | EmptyTank = 0 | 1
      | ManualReference between 0 and 1
      | Tempreature between 0 and 100
      | EmergencyButton = 0 | 1
      | LiquidLevel between 0 and 1 (hmax)
  note: Inputs For Tank2
  note: NAMES
      | --------------------------------------------
      | CT1 = ControlType Tank 1
      | F1 = Fill Tank 1
      | E1 = Empty Tank 1
      | MR1 = Manual Reference Tank1
      | T1 = Temperature Tank 1
      | EB1 = Emergency Button Tank 1
      | LL1 = Liquid Level 1
  note: Inputs For Tank3
  note: Inputs For Tank1
  CT1 : Inport
  T1 : Inport  Port=2
  EB1 : Inport  Port=3
  CT2 : Inport  Port=4
  F2 : Inport  Port=5
  E2 : Inport  Port=6
  MR2 : Inport  Port=7
  T2 : Inport  Port=8
  EB2 : Inport  Port=9
  CT3 : Inport  Port=10
  T3 : Inport  Port=11
  EB3 : Inport  Port=12
  Tank1 : Subsystem
  Tank2 : Subsystem
  Tank3 : Subsystem
  LL1 : Outport
  LL2 : Outport  Port=2
  LL3 : Outport  Port=3
  wires:
  EB1/1 -> Tank1/3(EB1)
  Tank2/1(LL2) -> LL2/1, Tank3/5(LL2), Tank1/4(LL2)
  Tank3/1(LL3) -> LL3/1, Tank2/8(LL3), Tank1/5(LL3)
  EB2/1 -> Tank2/6(EB2)
  CT2/1 -> Tank2/1(CT2)
  T1/1 -> Tank1/2(T1)
  Tank1/1(LL1) -> LL1/1, Tank3/4(LL1), Tank2/7(LL1)
  F2/1 -> Tank2/2(F2)
  E2/1 -> Tank2/3(E2)
  T2/1 -> Tank2/5(T2)
  CT3/1 -> Tank3/1(CT3)
  EB3/1 -> Tank3/3(EB3)
  T3/1 -> Tank3/2(T3)
  CT1/1 -> Tank1/1(CT1)
  MR2/1 -> Tank2/4(MR2)

== system c00013M_harness/M064 ==
  note: VALUES
      | ---------------------------------
      | ControlType = 1 | 2 | 3
      | FillTank = 0 | 1
      | EmptyTank = 0 | 1
      | ManualReference between 0 and 1
      | Tempreature between 0 and 100
      | EmergencyButton = 0 | 1
      | LiquidLevel between 0 and 1 (hmax)
  note: Inputs For Tank2
  note: NAMES
      | --------------------------------------------
      | CT1 = ControlType Tank 1
      | F1 = Fill Tank 1
      | E1 = Empty Tank 1
      | MR1 = Manual Reference Tank1
      | T1 = Temperature Tank 1
      | EB1 = Emergency Button Tank 1
      | LL1 = Liquid Level 1
  note: Inputs For Tank3
  note: Inputs For Tank1
  CT1 : Inport
  T1 : Inport  Port=2
  EB1 : Inport  Port=3
  CT2 : Inport  Port=4
  F2 : Inport  Port=5
  E2 : Inport  Port=6
  MR2 : Inport  Port=7
  T2 : Inport  Port=8
  EB2 : Inport  Port=9
  CT3 : Inport  Port=10
  T3 : Inport  Port=11
  EB3 : Inport  Port=12
  Tank1 : Subsystem
  Tank2 : Subsystem
  Tank3 : Subsystem
  LL1 : Outport
  LL2 : Outport  Port=2
  LL3 : Outport  Port=3
  wires:
  EB1/1 -> Tank1/3(EB1)
  Tank2/1(LL2) -> LL2/1, Tank3/5(LL2), Tank1/4(LL2)
  Tank3/1(LL3) -> LL3/1, Tank2/8(LL3), Tank1/5(LL3)
  EB2/1 -> Tank2/6(EB2)
  CT2/1 -> Tank2/1(CT2)
  T1/1 -> Tank1/2(T1)
  Tank1/1(LL1) -> LL1/1, Tank3/4(LL1), Tank2/7(LL1)
  F2/1 -> Tank2/2(F2)
  E2/1 -> Tank2/3(E2)
  T2/1 -> Tank2/5(T2)
  CT3/1 -> Tank3/1(CT3)
  EB3/1 -> Tank3/3(EB3)
  T3/1 -> Tank3/2(T3)
  CT1/1 -> Tank1/1(CT1)
  MR2/1 -> Tank2/4(MR2)

== system c00013M_harness/M065 ==
  note: VALUES
      | ---------------------------------
      | ControlType = 1 | 2 | 3
      | FillTank = 0 | 1
      | EmptyTank = 0 | 1
      | ManualReference between 0 and 1
      | Tempreature between 0 and 100
      | EmergencyButton = 0 | 1
      | LiquidLevel between 0 and 1 (hmax)
  note: Inputs For Tank2
  note: NAMES
      | --------------------------------------------
      | CT1 = ControlType Tank 1
      | F1 = Fill Tank 1
      | E1 = Empty Tank 1
      | MR1 = Manual Reference Tank1
      | T1 = Temperature Tank 1
      | EB1 = Emergency Button Tank 1
      | LL1 = Liquid Level 1
  note: Inputs For Tank3
  note: Inputs For Tank1
  CT1 : Inport
  T1 : Inport  Port=2
  EB1 : Inport  Port=3
  CT2 : Inport  Port=4
  F2 : Inport  Port=5
  E2 : Inport  Port=6
  MR2 : Inport  Port=7
  T2 : Inport  Port=8
  EB2 : Inport  Port=9
  CT3 : Inport  Port=10
  T3 : Inport  Port=11
  EB3 : Inport  Port=12
  Tank1 : Subsystem
  Tank2 : Subsystem
  Tank3 : Subsystem
  LL1 : Outport
  LL2 : Outport  Port=2
  LL3 : Outport  Port=3
  wires:
  EB1/1 -> Tank1/3(EB1)
  Tank2/1(LL2) -> LL2/1, Tank3/5(LL2), Tank1/4(LL2)
  Tank3/1(LL3) -> LL3/1, Tank2/8(LL3), Tank1/5(LL3)
  EB2/1 -> Tank2/6(EB2)
  CT2/1 -> Tank2/1(CT2)
  T1/1 -> Tank1/2(T1)
  Tank1/1(LL1) -> LL1/1, Tank3/4(LL1), Tank2/7(LL1)
  F2/1 -> Tank2/2(F2)
  E2/1 -> Tank2/3(E2)
  T2/1 -> Tank2/5(T2)
  CT3/1 -> Tank3/1(CT3)
  EB3/1 -> Tank3/3(EB3)
  T3/1 -> Tank3/2(T3)
  CT1/1 -> Tank1/1(CT1)
  MR2/1 -> Tank2/4(MR2)

== system c00013M_harness/M066 ==
  note: VALUES
      | ---------------------------------
      | ControlType = 1 | 2 | 3
      | FillTank = 0 | 1
      | EmptyTank = 0 | 1
      | ManualReference between 0 and 1
      | Tempreature between 0 and 100
      | EmergencyButton = 0 | 1
      | LiquidLevel between 0 and 1 (hmax)
  note: Inputs For Tank2
  note: NAMES
      | --------------------------------------------
      | CT1 = ControlType Tank 1
      | F1 = Fill Tank 1
      | E1 = Empty Tank 1
      | MR1 = Manual Reference Tank1
      | T1 = Temperature Tank 1
      | EB1 = Emergency Button Tank 1
      | LL1 = Liquid Level 1
  note: Inputs For Tank3
  note: Inputs For Tank1
  CT1 : Inport
  T1 : Inport  Port=2
  EB1 : Inport  Port=3
  CT2 : Inport  Port=4
  F2 : Inport  Port=5
  E2 : Inport  Port=6
  MR2 : Inport  Port=7
  T2 : Inport  Port=8
  EB2 : Inport  Port=9
  CT3 : Inport  Port=10
  T3 : Inport  Port=11
  EB3 : Inport  Port=12
  Tank1 : Subsystem
  Tank2 : Subsystem
  Tank3 : Subsystem
  LL1 : Outport
  LL2 : Outport  Port=2
  LL3 : Outport  Port=3
  wires:
  EB1/1 -> Tank1/3(EB1)
  Tank2/1(LL2) -> LL2/1, Tank3/5(LL2), Tank1/4(LL2)
  Tank3/1(LL3) -> LL3/1, Tank2/8(LL3), Tank1/5(LL3)
  EB2/1 -> Tank2/6(EB2)
  CT2/1 -> Tank2/1(CT2)
  T1/1 -> Tank1/2(T1)
  Tank1/1(LL1) -> LL1/1, Tank3/4(LL1), Tank2/7(LL1)
  F2/1 -> Tank2/2(F2)
  E2/1 -> Tank2/3(E2)
  T2/1 -> Tank2/5(T2)
  CT3/1 -> Tank3/1(CT3)
  EB3/1 -> Tank3/3(EB3)
  T3/1 -> Tank3/2(T3)
  CT1/1 -> Tank1/1(CT1)
  MR2/1 -> Tank2/4(MR2)

== system c00013M_harness/M067 ==
  note: VALUES
      | ---------------------------------
      | ControlType = 1 | 2 | 3
      | FillTank = 0 | 1
      | EmptyTank = 0 | 1
      | ManualReference between 0 and 1
      | Tempreature between 0 and 100
      | EmergencyButton = 0 | 1
      | LiquidLevel between 0 and 1 (hmax)
  note: Inputs For Tank2
  note: NAMES
      | --------------------------------------------
      | CT1 = ControlType Tank 1
      | F1 = Fill Tank 1
      | E1 = Empty Tank 1
      | MR1 = Manual Reference Tank1
      | T1 = Temperature Tank 1
      | EB1 = Emergency Button Tank 1
      | LL1 = Liquid Level 1
  note: Inputs For Tank3
  note: Inputs For Tank1
  CT1 : Inport
  T1 : Inport  Port=2
  EB1 : Inport  Port=3
  CT2 : Inport  Port=4
  F2 : Inport  Port=5
  E2 : Inport  Port=6
  MR2 : Inport  Port=7
  T2 : Inport  Port=8
  EB2 : Inport  Port=9
  CT3 : Inport  Port=10
  T3 : Inport  Port=11
  EB3 : Inport  Port=12
  Tank1 : Subsystem
  Tank2 : Subsystem
  Tank3 : Subsystem
  LL1 : Outport
  LL2 : Outport  Port=2
  LL3 : Outport  Port=3
  wires:
  EB1/1 -> Tank1/3(EB1)
  Tank2/1(LL2) -> LL2/1, Tank3/5(LL2), Tank1/4(LL2)
  Tank3/1(LL3) -> LL3/1, Tank2/8(LL3), Tank1/5(LL3)
  EB2/1 -> Tank2/6(EB2)
  CT2/1 -> Tank2/1(CT2)
  T1/1 -> Tank1/2(T1)
  Tank1/1(LL1) -> LL1/1, Tank3/4(LL1), Tank2/7(LL1)
  F2/1 -> Tank2/2(F2)
  E2/1 -> Tank2/3(E2)
  T2/1 -> Tank2/5(T2)
  CT3/1 -> Tank3/1(CT3)
  EB3/1 -> Tank3/3(EB3)
  T3/1 -> Tank3/2(T3)
  CT1/1 -> Tank1/1(CT1)
  MR2/1 -> Tank2/4(MR2)

== system c00013M_harness/M068 ==
  note: VALUES
      | ---------------------------------
      | ControlType = 1 | 2 | 3
      | FillTank = 0 | 1
      | EmptyTank = 0 | 1
      | ManualReference between 0 and 1
      | Tempreature between 0 and 100
      | EmergencyButton = 0 | 1
      | LiquidLevel between 0 and 1 (hmax)
  note: Inputs For Tank2
  note: NAMES
      | --------------------------------------------
      | CT1 = ControlType Tank 1
      | F1 = Fill Tank 1
      | E1 = Empty Tank 1
      | MR1 = Manual Reference Tank1
      | T1 = Temperature Tank 1
      | EB1 = Emergency Button Tank 1
      | LL1 = Liquid Level 1
  note: Inputs For Tank3
  note: Inputs For Tank1
  CT1 : Inport
  T1 : Inport  Port=2
  EB1 : Inport  Port=3
  CT2 : Inport  Port=4
  F2 : Inport  Port=5
  E2 : Inport  Port=6
  MR2 : Inport  Port=7
  T2 : Inport  Port=8
  EB2 : Inport  Port=9
  CT3 : Inport  Port=10
  T3 : Inport  Port=11
  EB3 : Inport  Port=12
  Tank1 : Subsystem
  Tank2 : Subsystem
  Tank3 : Subsystem
  LL1 : Outport
  LL2 : Outport  Port=2
  LL3 : Outport  Port=3
  wires:
  EB1/1 -> Tank1/3(EB1)
  Tank2/1(LL2) -> LL2/1, Tank3/5(LL2), Tank1/4(LL2)
  Tank3/1(LL3) -> LL3/1, Tank2/8(LL3), Tank1/5(LL3)
  EB2/1 -> Tank2/6(EB2)
  CT2/1 -> Tank2/1(CT2)
  T1/1 -> Tank1/2(T1)
  Tank1/1(LL1) -> LL1/1, Tank3/4(LL1), Tank2/7(LL1)
  F2/1 -> Tank2/2(F2)
  E2/1 -> Tank2/3(E2)
  T2/1 -> Tank2/5(T2)
  CT3/1 -> Tank3/1(CT3)
  EB3/1 -> Tank3/3(EB3)
  T3/1 -> Tank3/2(T3)
  CT1/1 -> Tank1/1(CT1)
  MR2/1 -> Tank2/4(MR2)

== system c00013M_harness/M069 ==
  note: VALUES
      | ---------------------------------
      | ControlType = 1 | 2 | 3
      | FillTank = 0 | 1
      | EmptyTank = 0 | 1
      | ManualReference between 0 and 1
      | Tempreature between 0 and 100
      | EmergencyButton = 0 | 1
      | LiquidLevel between 0 and 1 (hmax)
  note: Inputs For Tank2
  note: NAMES
      | --------------------------------------------
      | CT1 = ControlType Tank 1
      | F1 = Fill Tank 1
      | E1 = Empty Tank 1
      | MR1 = Manual Reference Tank1
      | T1 = Temperature Tank 1
      | EB1 = Emergency Button Tank 1
      | LL1 = Liquid Level 1
  note: Inputs For Tank3
  note: Inputs For Tank1
  CT1 : Inport
  T1 : Inport  Port=2
  EB1 : Inport  Port=3
  CT2 : Inport  Port=4
  F2 : Inport  Port=5
  E2 : Inport  Port=6
  MR2 : Inport  Port=7
  T2 : Inport  Port=8
  EB2 : Inport  Port=9
  CT3 : Inport  Port=10
  T3 : Inport  Port=11
  EB3 : Inport  Port=12
  Tank1 : Subsystem
  Tank2 : Subsystem
  Tank3 : Subsystem
  LL1 : Outport
  LL2 : Outport  Port=2
  LL3 : Outport  Port=3
  wires:
  EB1/1 -> Tank1/3(EB1)
  Tank2/1(LL2) -> LL2/1, Tank3/5(LL2), Tank1/4(LL2)
  Tank3/1(LL3) -> LL3/1, Tank2/8(LL3), Tank1/5(LL3)
  EB2/1 -> Tank2/6(EB2)
  CT2/1 -> Tank2/1(CT2)
  T1/1 -> Tank1/2(T1)
  Tank1/1(LL1) -> LL1/1, Tank3/4(LL1), Tank2/7(LL1)
  F2/1 -> Tank2/2(F2)
  E2/1 -> Tank2/3(E2)
  T2/1 -> Tank2/5(T2)
  CT3/1 -> Tank3/1(CT3)
  EB3/1 -> Tank3/3(EB3)
  T3/1 -> Tank3/2(T3)
  CT1/1 -> Tank1/1(CT1)
  MR2/1 -> Tank2/4(MR2)

== system c00013M_harness/M070 ==
  note: VALUES
      | ---------------------------------
      | ControlType = 1 | 2 | 3
      | FillTank = 0 | 1
      | EmptyTank = 0 | 1
      | ManualReference between 0 and 1
      | Tempreature between 0 and 100
      | EmergencyButton = 0 | 1
      | LiquidLevel between 0 and 1 (hmax)
  note: Inputs For Tank2
  note: NAMES
      | --------------------------------------------
      | CT1 = ControlType Tank 1
      | F1 = Fill Tank 1
      | E1 = Empty Tank 1
      | MR1 = Manual Reference Tank1
      | T1 = Temperature Tank 1
      | EB1 = Emergency Button Tank 1
      | LL1 = Liquid Level 1
  note: Inputs For Tank3
  note: Inputs For Tank1
  CT1 : Inport
  T1 : Inport  Port=2
  EB1 : Inport  Port=3
  CT2 : Inport  Port=4
  F2 : Inport  Port=5
  E2 : Inport  Port=6
  MR2 : Inport  Port=7
  T2 : Inport  Port=8
  EB2 : Inport  Port=9
  CT3 : Inport  Port=10
  T3 : Inport  Port=11
  EB3 : Inport  Port=12
  Tank1 : Subsystem
  Tank2 : Subsystem
  Tank3 : Subsystem
  LL1 : Outport
  LL2 : Outport  Port=2
  LL3 : Outport  Port=3
  wires:
  EB1/1 -> Tank1/3(EB1)
  Tank2/1(LL2) -> LL2/1, Tank3/5(LL2), Tank1/4(LL2)
  Tank3/1(LL3) -> LL3/1, Tank2/8(LL3), Tank1/5(LL3)
  EB2/1 -> Tank2/6(EB2)
  CT2/1 -> Tank2/1(CT2)
  T1/1 -> Tank1/2(T1)
  Tank1/1(LL1) -> LL1/1, Tank3/4(LL1), Tank2/7(LL1)
  F2/1 -> Tank2/2(F2)
  E2/1 -> Tank2/3(E2)
  T2/1 -> Tank2/5(T2)
  CT3/1 -> Tank3/1(CT3)
  EB3/1 -> Tank3/3(EB3)
  T3/1 -> Tank3/2(T3)
  CT1/1 -> Tank1/1(CT1)
  MR2/1 -> Tank2/4(MR2)

== system c00013M_harness/M071 ==
  note: VALUES
      | ---------------------------------
      | ControlType = 1 | 2 | 3
      | FillTank = 0 | 1
      | EmptyTank = 0 | 1
      | ManualReference between 0 and 1
      | Tempreature between 0 and 100
      | EmergencyButton = 0 | 1
      | LiquidLevel between 0 and 1 (hmax)
  note: Inputs For Tank2
  note: NAMES
      | --------------------------------------------
      | CT1 = ControlType Tank 1
      | F1 = Fill Tank 1
      | E1 = Empty Tank 1
      | MR1 = Manual Reference Tank1
      | T1 = Temperature Tank 1
      | EB1 = Emergency Button Tank 1
      | LL1 = Liquid Level 1
  note: Inputs For Tank3
  note: Inputs For Tank1
  CT1 : Inport
  T1 : Inport  Port=2
  EB1 : Inport  Port=3
  CT2 : Inport  Port=4
  F2 : Inport  Port=5
  E2 : Inport  Port=6
  MR2 : Inport  Port=7
  T2 : Inport  Port=8
  EB2 : Inport  Port=9
  CT3 : Inport  Port=10
  T3 : Inport  Port=11
  EB3 : Inport  Port=12
  Tank1 : Subsystem
  Tank2 : Subsystem
  Tank3 : Subsystem
  LL1 : Outport
  LL2 : Outport  Port=2
  LL3 : Outport  Port=3
  wires:
  EB1/1 -> Tank1/3(EB1)
  Tank2/1(LL2) -> LL2/1, Tank3/5(LL2), Tank1/4(LL2)
  Tank3/1(LL3) -> LL3/1, Tank2/8(LL3), Tank1/5(LL3)
  EB2/1 -> Tank2/6(EB2)
  CT2/1 -> Tank2/1(CT2)
  T1/1 -> Tank1/2(T1)
  Tank1/1(LL1) -> LL1/1, Tank3/4(LL1), Tank2/7(LL1)
  F2/1 -> Tank2/2(F2)
  E2/1 -> Tank2/3(E2)
  T2/1 -> Tank2/5(T2)
  CT3/1 -> Tank3/1(CT3)
  EB3/1 -> Tank3/3(EB3)
  T3/1 -> Tank3/2(T3)
  CT1/1 -> Tank1/1(CT1)
  MR2/1 -> Tank2/4(MR2)

== system c00013M_harness/M072 ==
  note: VALUES
      | ---------------------------------
      | ControlType = 1 | 2 | 3
      | FillTank = 0 | 1
      | EmptyTank = 0 | 1
      | ManualReference between 0 and 1
      | Tempreature between 0 and 100
      | EmergencyButton = 0 | 1
      | LiquidLevel between 0 and 1 (hmax)
  note: Inputs For Tank2
  note: NAMES
      | --------------------------------------------
      | CT1 = ControlType Tank 1
      | F1 = Fill Tank 1
      | E1 = Empty Tank 1
      | MR1 = Manual Reference Tank1
      | T1 = Temperature Tank 1
      | EB1 = Emergency Button Tank 1
      | LL1 = Liquid Level 1
  note: Inputs For Tank3
  note: Inputs For Tank1
  CT1 : Inport
  T1 : Inport  Port=2
  EB1 : Inport  Port=3
  CT2 : Inport  Port=4
  F2 : Inport  Port=5
  E2 : Inport  Port=6
  MR2 : Inport  Port=7
  T2 : Inport  Port=8
  EB2 : Inport  Port=9
  CT3 : Inport  Port=10
  T3 : Inport  Port=11
  EB3 : Inport  Port=12
  Tank1 : Subsystem
  Tank2 : Subsystem
  Tank3 : Subsystem
  LL1 : Outport
  LL2 : Outport  Port=2
  LL3 : Outport  Port=3
  wires:
  EB1/1 -> Tank1/3(EB1)
  Tank2/1(LL2) -> LL2/1, Tank3/5(LL2), Tank1/4(LL2)
  Tank3/1(LL3) -> LL3/1, Tank2/8(LL3), Tank1/5(LL3)
  EB2/1 -> Tank2/6(EB2)
  CT2/1 -> Tank2/1(CT2)
  T1/1 -> Tank1/2(T1)
  Tank1/1(LL1) -> LL1/1, Tank3/4(LL1), Tank2/7(LL1)
  F2/1 -> Tank2/2(F2)
  E2/1 -> Tank2/3(E2)
  T2/1 -> Tank2/5(T2)
  CT3/1 -> Tank3/1(CT3)
  EB3/1 -> Tank3/3(EB3)
  T3/1 -> Tank3/2(T3)
  CT1/1 -> Tank1/1(CT1)
  MR2/1 -> Tank2/4(MR2)

== system c00013M_harness/M073 ==
  note: VALUES
      | ---------------------------------
      | ControlType = 1 | 2 | 3
      | FillTank = 0 | 1
      | EmptyTank = 0 | 1
      | ManualReference between 0 and 1
      | Tempreature between 0 and 100
      | EmergencyButton = 0 | 1
      | LiquidLevel between 0 and 1 (hmax)
  note: Inputs For Tank2
  note: NAMES
      | --------------------------------------------
      | CT1 = ControlType Tank 1
      | F1 = Fill Tank 1
      | E1 = Empty Tank 1
      | MR1 = Manual Reference Tank1
      | T1 = Temperature Tank 1
      | EB1 = Emergency Button Tank 1
      | LL1 = Liquid Level 1
  note: Inputs For Tank3
  note: Inputs For Tank1
  CT1 : Inport
  T1 : Inport  Port=2
  EB1 : Inport  Port=3
  CT2 : Inport  Port=4
  F2 : Inport  Port=5
  E2 : Inport  Port=6
  MR2 : Inport  Port=7
  T2 : Inport  Port=8
  EB2 : Inport  Port=9
  CT3 : Inport  Port=10
  T3 : Inport  Port=11
  EB3 : Inport  Port=12
  Tank1 : Subsystem
  Tank2 : Subsystem
  Tank3 : Subsystem
  LL1 : Outport
  LL2 : Outport  Port=2
  LL3 : Outport  Port=3
  wires:
  EB1/1 -> Tank1/3(EB1)
  Tank2/1(LL2) -> LL2/1, Tank3/5(LL2), Tank1/4(LL2)
  Tank3/1(LL3) -> LL3/1, Tank2/8(LL3), Tank1/5(LL3)
  EB2/1 -> Tank2/6(EB2)
  CT2/1 -> Tank2/1(CT2)
  T1/1 -> Tank1/2(T1)
  Tank1/1(LL1) -> LL1/1, Tank3/4(LL1), Tank2/7(LL1)
  F2/1 -> Tank2/2(F2)
  E2/1 -> Tank2/3(E2)
  T2/1 -> Tank2/5(T2)
  CT3/1 -> Tank3/1(CT3)
  EB3/1 -> Tank3/3(EB3)
  T3/1 -> Tank3/2(T3)
  CT1/1 -> Tank1/1(CT1)
  MR2/1 -> Tank2/4(MR2)

== system c00013M_harness/M074 ==
  note: VALUES
      | ---------------------------------
      | ControlType = 1 | 2 | 3
      | FillTank = 0 | 1
      | EmptyTank = 0 | 1
      | ManualReference between 0 and 1
      | Tempreature between 0 and 100
      | EmergencyButton = 0 | 1
      | LiquidLevel between 0 and 1 (hmax)
  note: Inputs For Tank2
  note: NAMES
      | --------------------------------------------
      | CT1 = ControlType Tank 1
      | F1 = Fill Tank 1
      | E1 = Empty Tank 1
      | MR1 = Manual Reference Tank1
      | T1 = Temperature Tank 1
      | EB1 = Emergency Button Tank 1
      | LL1 = Liquid Level 1
  note: Inputs For Tank3
  note: Inputs For Tank1
  CT1 : Inport
  T1 : Inport  Port=2
  EB1 : Inport  Port=3
  CT2 : Inport  Port=4
  F2 : Inport  Port=5
  E2 : Inport  Port=6
  MR2 : Inport  Port=7
  T2 : Inport  Port=8
  EB2 : Inport  Port=9
  CT3 : Inport  Port=10
  T3 : Inport  Port=11
  EB3 : Inport  Port=12
  Tank1 : Subsystem
  Tank2 : Subsystem
  Tank3 : Subsystem
  LL1 : Outport
  LL2 : Outport  Port=2
  LL3 : Outport  Port=3
  wires:
  EB1/1 -> Tank1/3(EB1)
  Tank2/1(LL2) -> LL2/1, Tank3/5(LL2), Tank1/4(LL2)
  Tank3/1(LL3) -> LL3/1, Tank2/8(LL3), Tank1/5(LL3)
  EB2/1 -> Tank2/6(EB2)
  CT2/1 -> Tank2/1(CT2)
  T1/1 -> Tank1/2(T1)
  Tank1/1(LL1) -> LL1/1, Tank3/4(LL1), Tank2/7(LL1)
  F2/1 -> Tank2/2(F2)
  E2/1 -> Tank2/3(E2)
  T2/1 -> Tank2/5(T2)
  CT3/1 -> Tank3/1(CT3)
  EB3/1 -> Tank3/3(EB3)
  T3/1 -> Tank3/2(T3)
  CT1/1 -> Tank1/1(CT1)
  MR2/1 -> Tank2/4(MR2)

== system c00013M_harness/M075 ==
  note: VALUES
      | ---------------------------------
      | ControlType = 1 | 2 | 3
      | FillTank = 0 | 1
      | EmptyTank = 0 | 1
      | ManualReference between 0 and 1
      | Tempreature between 0 and 100
      | EmergencyButton = 0 | 1
      | LiquidLevel between 0 and 1 (hmax)
  note: Inputs For Tank2
  note: NAMES
      | --------------------------------------------
      | CT1 = ControlType Tank 1
      | F1 = Fill Tank 1
      | E1 = Empty Tank 1
      | MR1 = Manual Reference Tank1
      | T1 = Temperature Tank 1
      | EB1 = Emergency Button Tank 1
      | LL1 = Liquid Level 1
  note: Inputs For Tank3
  note: Inputs For Tank1
  CT1 : Inport
  T1 : Inport  Port=2
  EB1 : Inport  Port=3
  CT2 : Inport  Port=4
  F2 : Inport  Port=5
  E2 : Inport  Port=6
  MR2 : Inport  Port=7
  T2 : Inport  Port=8
  EB2 : Inport  Port=9
  CT3 : Inport  Port=10
  T3 : Inport  Port=11
  EB3 : Inport  Port=12
  Tank1 : Subsystem
  Tank2 : Subsystem
  Tank3 : Subsystem
  LL1 : Outport
  LL2 : Outport  Port=2
  LL3 : Outport  Port=3
  wires:
  EB1/1 -> Tank1/3(EB1)
  Tank2/1(LL2) -> LL2/1, Tank3/5(LL2), Tank1/4(LL2)
  Tank3/1(LL3) -> LL3/1, Tank2/8(LL3), Tank1/5(LL3)
  EB2/1 -> Tank2/6(EB2)
  CT2/1 -> Tank2/1(CT2)
  T1/1 -> Tank1/2(T1)
  Tank1/1(LL1) -> LL1/1, Tank3/4(LL1), Tank2/7(LL1)
  F2/1 -> Tank2/2(F2)
  E2/1 -> Tank2/3(E2)
  T2/1 -> Tank2/5(T2)
  CT3/1 -> Tank3/1(CT3)
  EB3/1 -> Tank3/3(EB3)
  T3/1 -> Tank3/2(T3)
  CT1/1 -> Tank1/1(CT1)
  MR2/1 -> Tank2/4(MR2)

== system c00013M_harness/M076 ==
  note: VALUES
      | ---------------------------------
      | ControlType = 1 | 2 | 3
      | FillTank = 0 | 1
      | EmptyTank = 0 | 1
      | ManualReference between 0 and 1
      | Tempreature between 0 and 100
      | EmergencyButton = 0 | 1
      | LiquidLevel between 0 and 1 (hmax)
  note: Inputs For Tank2
  note: NAMES
      | --------------------------------------------
      | CT1 = ControlType Tank 1
      | F1 = Fill Tank 1
      | E1 = Empty Tank 1
      | MR1 = Manual Reference Tank1
      | T1 = Temperature Tank 1
      | EB1 = Emergency Button Tank 1
      | LL1 = Liquid Level 1
  note: Inputs For Tank3
  note: Inputs For Tank1
  CT1 : Inport
  T1 : Inport  Port=2
  EB1 : Inport  Port=3
  CT2 : Inport  Port=4
  F2 : Inport  Port=5
  E2 : Inport  Port=6
  MR2 : Inport  Port=7
  T2 : Inport  Port=8
  EB2 : Inport  Port=9
  CT3 : Inport  Port=10
  T3 : Inport  Port=11
  EB3 : Inport  Port=12
  Tank1 : Subsystem
  Tank2 : Subsystem
  Tank3 : Subsystem
  LL1 : Outport
  LL2 : Outport  Port=2
  LL3 : Outport  Port=3
  wires:
  EB1/1 -> Tank1/3(EB1)
  Tank2/1(LL2) -> LL2/1, Tank3/5(LL2), Tank1/4(LL2)
  Tank3/1(LL3) -> LL3/1, Tank2/8(LL3), Tank1/5(LL3)
  EB2/1 -> Tank2/6(EB2)
  CT2/1 -> Tank2/1(CT2)
  T1/1 -> Tank1/2(T1)
  Tank1/1(LL1) -> LL1/1, Tank3/4(LL1), Tank2/7(LL1)
  F2/1 -> Tank2/2(F2)
  E2/1 -> Tank2/3(E2)
  T2/1 -> Tank2/5(T2)
  CT3/1 -> Tank3/1(CT3)
  EB3/1 -> Tank3/3(EB3)
  T3/1 -> Tank3/2(T3)
  CT1/1 -> Tank1/1(CT1)
  MR2/1 -> Tank2/4(MR2)

== system c00013M_harness/M077 ==
  note: VALUES
      | ---------------------------------
      | ControlType = 1 | 2 | 3
      | FillTank = 0 | 1
      | EmptyTank = 0 | 1
      | ManualReference between 0 and 1
      | Tempreature between 0 and 100
      | EmergencyButton = 0 | 1
      | LiquidLevel between 0 and 1 (hmax)
  note: Inputs For Tank2
  note: NAMES
      | --------------------------------------------
      | CT1 = ControlType Tank 1
      | F1 = Fill Tank 1
      | E1 = Empty Tank 1
      | MR1 = Manual Reference Tank1
      | T1 = Temperature Tank 1
      | EB1 = Emergency Button Tank 1
      | LL1 = Liquid Level 1
  note: Inputs For Tank3
  note: Inputs For Tank1
  CT1 : Inport
  T1 : Inport  Port=2
  EB1 : Inport  Port=3
  CT2 : Inport  Port=4
  F2 : Inport  Port=5
  E2 : Inport  Port=6
  MR2 : Inport  Port=7
  T2 : Inport  Port=8
  EB2 : Inport  Port=9
  CT3 : Inport  Port=10
  T3 : Inport  Port=11
  EB3 : Inport  Port=12
  Tank1 : Subsystem
  Tank2 : Subsystem
  Tank3 : Subsystem
  LL1 : Outport
  LL2 : Outport  Port=2
  LL3 : Outport  Port=3
  wires:
  EB1/1 -> Tank1/3(EB1)
  Tank2/1(LL2) -> LL2/1, Tank3/5(LL2), Tank1/4(LL2)
  Tank3/1(LL3) -> LL3/1, Tank2/8(LL3), Tank1/5(LL3)
  EB2/1 -> Tank2/6(EB2)
  CT2/1 -> Tank2/1(CT2)
  T1/1 -> Tank1/2(T1)
  Tank1/1(LL1) -> LL1/1, Tank3/4(LL1), Tank2/7(LL1)
  F2/1 -> Tank2/2(F2)
  E2/1 -> Tank2/3(E2)
  T2/1 -> Tank2/5(T2)
  CT3/1 -> Tank3/1(CT3)
  EB3/1 -> Tank3/3(EB3)
  T3/1 -> Tank3/2(T3)
  CT1/1 -> Tank1/1(CT1)
  MR2/1 -> Tank2/4(MR2)
